simulink model "RobotSimParking"  (R2024b)
settings: Solver=FixedStepAuto  StartTime=0.0  StopTime=15  FixedStep=0.02  RelTol=1e-3
values from neighbouring files (symbols this model uses):
  l = robot_params(2)    [transformationMatrix.m]
undefined symbols (not defined in the file or in its folder): DiscIntNeverNeededParam, robot_params, Ts
settings Model: Creator=fabio  LastModifiedBy=felip
settings SolverCC: AlgebraicLoopSolver=TrustRegion
settings OptimizationCC: BlockReduction=off  DefaultParameterBehavior=Inlined  BufferReuse=off
settings DebuggingCC: UnconnectedInputMsg=warning  UnconnectedOutputMsg=warning  UnconnectedLineMsg=warning
settings ModelReferenceCC: EnableRefExpFcnMdlSchedulingChecks=on
settings RTWCC: GPUComputeCapability=3.5  DLArmComputeVersion=19.05

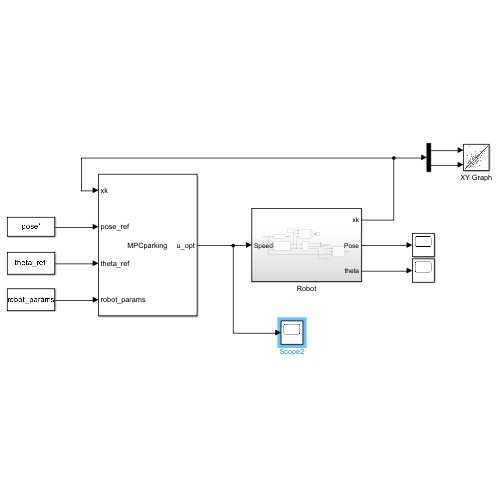
[thumbnail: Simulink's stored preview of the top-level diagram]
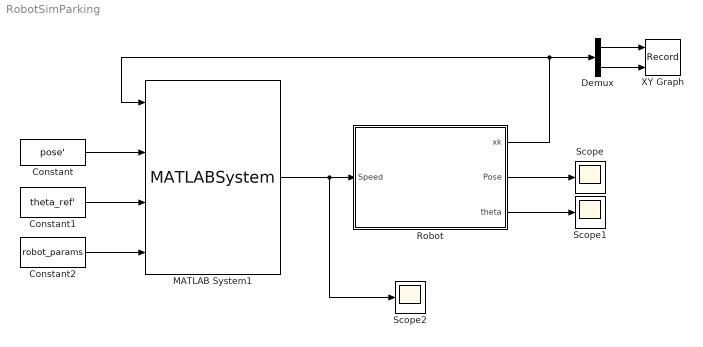
== system RobotSimParking ==
  Constant : Constant  Value=pose'  SampleTime=Ts
  Constant1 : Constant  Value=theta_ref'  SampleTime=Ts
  Constant2 : Constant  Value=robot_params
  Demux : Demux  Outputs=2
  MATLAB System1 : MATLABSystem  System=MPCparking  tau_s=0.2  Q=10*eye(2)  R=2*eye(2)  P=12*eye(2)  Y=3*eye(2)  N=10  epsilon=0.3  SimulateUsing=Interpreted execution
      mask Type: MPCparking
      mask Display:
      | disp('MPCparking');
      | port_label('input',1,'xk');
      | port_label('input',2,'pose_ref');
      | port_label('input',3,'theta_ref');
      | port_label('input',4,'robot_params');
      | port_label('output',1,'u_opt');
  Robot : Subsystem
  Scope : Scope
  Scope1 : Scope
  Scope2 : Scope
  XY Graph : Record  FileSettingsInternal="{\"entries\":[{\"content\":{\"excelSettings\":{\"content\":{},\"type\":\"Streamout.ExcelSettings\"}},\"type\":\"Streamout.FileSettingStorage\",\"uuid\":\"\"}],\"packageUris\":[\"http:\\/\\/schema.mathworks.com\\/mf0\\/streamout_blocks\\/R2020a\"],\"version\":\"1.0\"}"  Layout=[1 1]  SignalsInternal="{\"entries\":[{\"content\":{\"signals\":[{\"content\":{\"blockPath\":[],\"dimensions\":[1,1],\"domain\":\"\",\"lineColor\":\"#a2142f\",\"plots\":[ 1 ],\"port\":1,\"sid\":[\"\"],\"signalID\":1,\"signalName\":\"Demux:1\"},\"type\":\"RecordBlkView.Signal\",\"uuid\":\"\"},{\"content\":{\"blockPath\":[],\"dimensions\":[1,1],\"domain\":\"\",\"lineColor\":\"#139fff\",\"plots\":[ 1 ],\"port\":2,\"sid\":[\"\"],\"signalID\":2,\"signalName\":\"Demux:2\"},\"type\":\"RecordBlkView.Signal\",\"uuid\":\"\"}]},\"type\":\"RecordBlkView.InputSignals\",\"uuid\":\"\"}],\"packageUris\":[\"http:\\/\\/schema.mathworks.com\\/mf0\\/streamout_blocks\\/R2020a\"],\"version\":\"1.0\"}"  VisualizationBindings="{\"xyplotplugin\":{\"info\":[{\"series\":[{\"bindingParametersList\":[{\"parameter\":\"X-Axis\",\"signalID\":1,\"signalName\":\"Demux:1\"},{\"parameter\":\"Y-Axis\",\"signalID\":2,\"signalName\":\"Demux:2\"}],\"seriesID\":0}],\"subplotID\":1}]}}"  CompatibilityTag=XY
  wires:
  MATLAB System1/1 -> Scope2/1, Robot/1(Speed)
  Robot/2(Pose) -> Scope/1
  Robot/3(theta) -> Scope1/1
  Constant/1 -> MATLAB System1/2
  Constant1/1 -> MATLAB System1/3
  Demux/1 -> XY Graph/1
  Demux/2 -> XY Graph/2
  Robot/1(xk) -> MATLAB System1/1, Demux/1
  Constant2/1 -> MATLAB System1/4

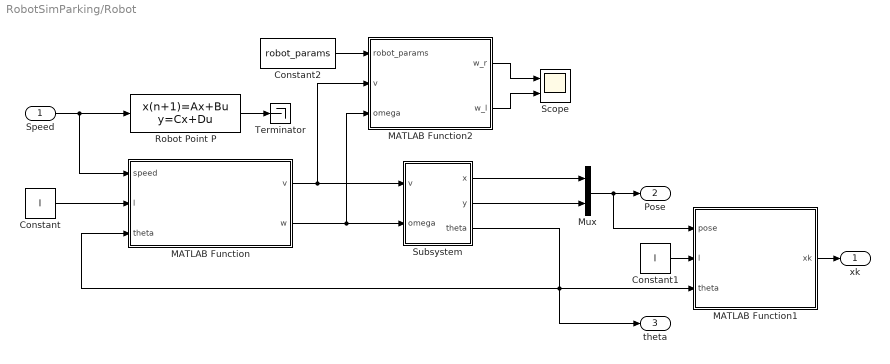
== system RobotSimParking/Robot ==
  Speed : Inport
  Constant : Constant  Value=l
  Constant1 : Constant  Value=l
  Constant2 : Constant  Value=robot_params
  MATLAB Function : MATLAB Function  TreatAsAtomicUnit=on
  MATLAB Function1 : MATLAB Function  TreatAsAtomicUnit=on
  MATLAB Function2 : MATLAB Function  TreatAsAtomicUnit=on
  Mux : Mux  Inputs=2
  Robot Point P : DiscreteStateSpace  A=eye(2)  B=Ts*eye(2)  C=eye(2)  D=zeros(2)  InitialCondition=zeros(2,1)  SampleTime=Ts
  Scope : Scope  NumInputPorts=2
  Subsystem : Subsystem
  Terminator : Terminator
  xk : Outport
  Pose : Outport  Port=2
  theta : Outport  Port=3
  wires:
  Speed/1 -> Robot Point P/1, MATLAB Function/1(speed)
  Constant/1 -> MATLAB Function/2(l)
  Subsystem/3(theta) -> MATLAB Function/3(theta), theta/1, MATLAB Function1/3(theta)
  MATLAB Function/1(v) -> MATLAB Function2/2(v), Subsystem/1(v)
  MATLAB Function/2(w) -> MATLAB Function2/3(omega), Subsystem/2(omega)
  Subsystem/1(x) -> Mux/1
  Subsystem/2(y) -> Mux/2
  Mux/1 -> Pose/1, MATLAB Function1/1(pose)
  Constant1/1 -> MATLAB Function1/2(l)
  MATLAB Function1/1(xk) -> xk/1
  Robot Point P/1 -> Terminator/1
  Constant2/1 -> MATLAB Function2/1(robot_params)
  MATLAB Function2/1(w_r) -> Scope/1
  MATLAB Function2/2(w_l) -> Scope/2

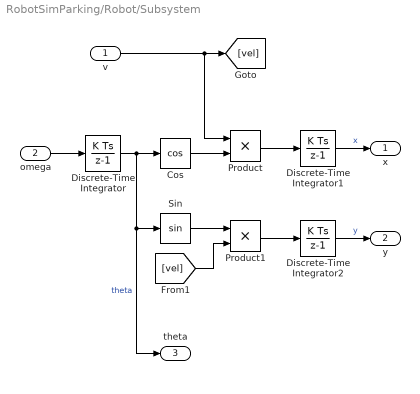
== system RobotSimParking/Robot/Subsystem ==
  v : Inport
  omega : Inport  Port=2
  Cos : Trigonometry  Operator=cos
  Discrete-Time Integrator : DiscreteIntegrator  SampleTime=0.02  ICPrevOutput=DiscIntNeverNeededParam  ICPrevScaledInput=DiscIntNeverNeededParam
  Discrete-Time Integrator1 : DiscreteIntegrator  InitialCondition=-1  SampleTime=0.02  ICPrevOutput=DiscIntNeverNeededParam  ICPrevScaledInput=DiscIntNeverNeededParam
  Discrete-Time Integrator2 : DiscreteIntegrator  SampleTime=0.02  ICPrevOutput=DiscIntNeverNeededParam  ICPrevScaledInput=DiscIntNeverNeededParam
  Product : Product
  Product1 : Product
  Sin : Trigonometry
  x : Outport
  y : Outport  Port=2
  theta : Outport  Port=3
  wires:
  Product1/1 -> Discrete-Time Integrator2/1
  Cos/1 -> Product/2
  Product/1 -> Discrete-Time Integrator1/1
  omega/1 -> Discrete-Time Integrator/1
  Discrete-Time Integrator1/1 -> x/1  "x"
  Discrete-Time Integrator2/1 -> y/1  "y"
  Discrete-Time Integrator/1 -> theta/1, Sin/1, Cos/1  "theta"
  v/1 -> Product/1, [vel]
  Sin/1 -> Product1/1
  [vel] -> Product1/2

== matlab function RobotSimParking/Robot/MATLAB Function1 ==
  data: pose input; xk output; l input; theta input
function xk = transformationToP(pose, l, theta)
xk = zeros(2,1);
xk = [pose(1) + l*cos(theta), pose(2) + l*sin(theta)]';

== matlab function RobotSimParking/Robot/MATLAB Function ==
  data: speed input; v output; l input; theta input; w output
function [v,w] = Transformation(speed, l, theta)
    % theta: heading angle
    % l: distance to point p

    T = [cos(theta) -l*sin(theta);
         sin(theta) l*cos(theta)];

    anti = T\speed;
    
    v = anti(1);
    w = anti(2);

== matlab function RobotSimParking/Robot/MATLAB Function2 ==
  data: robot_params input; v input; w_r output; omega input; w_l output
function [w_r, w_l] = w_wheels(robot_params, v, omega)
R = robot_params(3);
L = robot_params(1);
omegas = (1/R)*[1 L/2; 1 -L/2]*[v omega]';
w_r = omegas(1);
w_l = omegas(2);
